simulink model "PD_SMC"  (R2017b)
settings: Solver=FixedStepAuto  StartTime=0.0  StopTime=100  FixedStep=0.01  RelTol=1e-3
values from neighbouring files (symbols this model uses):
  g = 9.81    [matlab.mat]    (also in thongsohethong.m = 9.8)
  L = 0.3    [thongsohethong.m]
  Mb = 7    [thongsohethong.m]
  Mw = 0.03    [matlab.mat]    (also in thongsohethong.m = 0.5)
  R = 1    [matlab.mat]    (also in thongsohethong.m = 0.07)
settings Model: Creator=DELL  LastModifiedBy=DELL

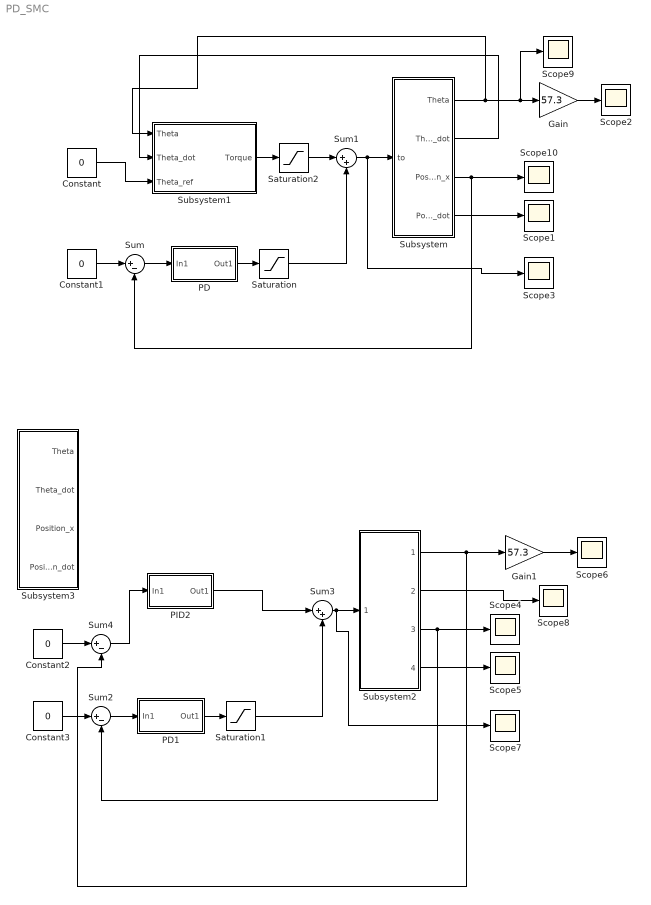
== system PD_SMC ==
  Constant{,1..3} (4 alike) : Constant  Value=0
  Gain : Gain  Gain=57.3
  Gain1 : Gain  Gain=57.3
  PD : Subsystem
  PD1 : Subsystem
  PID2 : Subsystem
  Saturation : Saturate  UpperLimit=0.25  LowerLimit=-0.25
  Saturation1 : Saturate
  Saturation2 : Saturate  UpperLimit=0.75  LowerLimit=-0.75
  Scope{1..10} (10 alike) : Scope
  Subsystem : Subsystem
  Subsystem1 : Subsystem
  Subsystem2 : Subsystem
  Subsystem3 : Subsystem
  Sum : Sum  Inputs=|+-
  Sum1 : Sum  Inputs=|++
  Sum2 : Sum  Inputs=|+-
  Sum3 : Sum  Inputs=|++
  Sum4 : Sum  Inputs=|+-
  wires:
  Subsystem/1(Theta) -> Subsystem1/1(Theta), Scope9/1, Gain/1
  Subsystem/2(Theta_dot) -> Subsystem1/2(Theta_dot)
  Subsystem/3(Position_x) -> Scope10/1, Sum/2
  Subsystem/4(Position_dot) -> Scope1/1
  Constant/1 -> Subsystem1/3(Theta_ref)
  Constant1/1 -> Sum/1
  Sum/1 -> PD/1(In1)
  PD/1(Out1) -> Saturation/1
  Saturation/1 -> Sum1/2
  Gain/1 -> Scope2/1
  Subsystem1/1(Torque) -> Saturation2/1
  PID2/1(Out1) -> Sum3/1
  PD1/1(Out1) -> Saturation1/1
  Sum2/1 -> PD1/1(In1)
  Sum3/1 -> Scope7/1, Subsystem2/1(Moment_motor)
  Constant3/1 -> Sum2/1
  Subsystem2/4(Position_dot) -> Scope5/1
  Subsystem2/1(Theta) -> Sum4/2, Gain1/1
  Saturation1/1 -> Sum3/2
  Subsystem2/3(Position_x) -> Sum2/2, Scope4/1
  Gain1/1 -> Scope6/1
  Constant2/1 -> Sum4/1
  Sum4/1 -> PID2/1(In1)
  Subsystem2/2(Theta_dot) -> Scope8/1
  Sum1/1 -> Scope3/1, Subsystem/1(to)
  Saturation2/1 -> Sum1/1

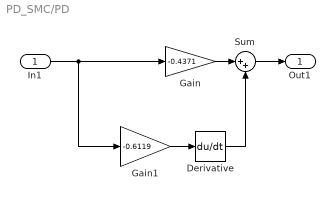
== system PD_SMC/PD ==
  In1 : Inport
  Derivative : Derivative
  Gain : Gain  Gain=-0.4371
  Gain1 : Gain  Gain=-0.6119
  Sum : Sum  Inputs=|++
  Out1 : Outport
  wires:
  In1/1 -> Gain1/1, Gain/1
  Gain1/1 -> Derivative/1
  Gain/1 -> Sum/1
  Sum/1 -> Out1/1
  Derivative/1 -> Sum/2

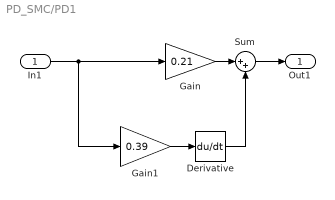
== system PD_SMC/PD1 ==
  In1 : Inport
  Derivative : Derivative
  Gain : Gain  Gain=0.21
  Gain1 : Gain  Gain=0.39
  Sum : Sum  Inputs=|++
  Out1 : Outport
  wires:
  In1/1 -> Gain1/1, Gain/1
  Gain1/1 -> Derivative/1
  Gain/1 -> Sum/1
  Sum/1 -> Out1/1
  Derivative/1 -> Sum/2

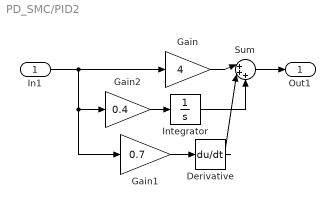
== system PD_SMC/PID2 ==
  In1 : Inport
  Derivative : Derivative
  Gain : Gain  Gain=4
  Gain1 : Gain  Gain=0.7
  Gain2 : Gain  Gain=0.4
  Integrator : Integrator
  Sum : Sum  Inputs=|+++
  Out1 : Outport
  wires:
  Derivative/1 -> Sum/2
  Sum/1 -> Out1/1
  Gain/1 -> Sum/1
  Gain1/1 -> Derivative/1
  In1/1 -> Gain/1, Gain2/1, Gain1/1
  Gain2/1 -> Integrator/1
  Integrator/1 -> Sum/3

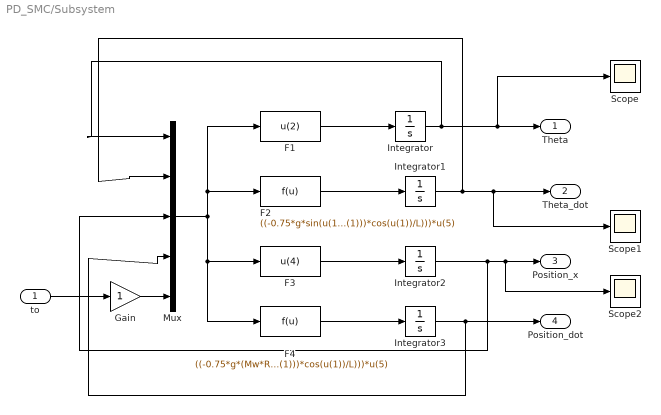
== system PD_SMC/Subsystem ==
  to : Inport
  F1 : Fcn  Expr=u(2)
  F2 : Fcn  Expr=((-0.75*g*sin(u(1))/L)/((0.75*((Mw*R+Mb*L*cos(u(1)))*cos(u(1)))/(2*Mw+Mb)*L)-1))+((0.75*Mb*L*sin(u(1))*cos(u(1))*(u(2)^2)/(2*Mw+Mb)*L)/((0.75*(Mw*R+Mb*L*cos(u(1)))*cos(u(1))/(2*Mw+Mb)*L)-1))+(((0.75*(Mw*R+Mb*L*cos(u(1)))*(1+(sin(u(1))^2)))+1/R)/(2*Mw+Mb-(0.75*(Mw*R+Mb*L*cos(u(1)))*cos(u(1))/L)))*u(5)
  F3 : Fcn  Expr=u(4)
  F4 : Fcn  Expr=((-0.75*g*(Mw*R+Mb*L*cos(u(1)))*sin(u(1)))/(2*Mw+Mb-(0.75*(Mw*R+Mb*L*cos(u(1)))*cos(u(1))/L)))+((Mb*L*sin(u(1))*(u(2)^2))/(2*Mw+Mb-(0.75*(Mw*R+Mb*L*cos(u(1)))*cos(u(1))/L)))+((0.75*(Mw*R+Mb*L*cos(u(1)))*(1+(sin(u(1))^2))+1/R)/(Mb*L^2)+(1/R)/(2*Mw+Mb-(0.75*(Mw*R+Mb*L*cos(u(1)))*cos(u(1))/L)))*u(5)
  Gain : Gain
  Integrator : Integrator  InitialCondition=0.3
  Integrator1 : Integrator
  Integrator2 : Integrator
  Integrator3 : Integrator
  Mux : Mux  Inputs=5
  Scope : Scope
  Scope1 : Scope
  Scope2 : Scope
  Theta : Outport
  Theta_dot : Outport  Port=2
  Position_x : Outport  Port=3
  Position_dot : Outport  Port=4
  wires:
  Gain/1 -> Mux/5
  F4/1 -> Integrator3/1
  Integrator3/1 -> Position_dot/1, Mux/4
  Integrator2/1 -> Mux/3, Position_x/1, Scope2/1
  Integrator/1 -> Theta/1, Scope/1, Mux/1
  F3/1 -> Integrator2/1
  F1/1 -> Integrator/1
  F2/1 -> Integrator1/1
  Integrator1/1 -> Theta_dot/1, Scope1/1, Mux/2
  Mux/1 -> F4/1, F3/1, F2/1, F1/1
  to/1 -> Gain/1

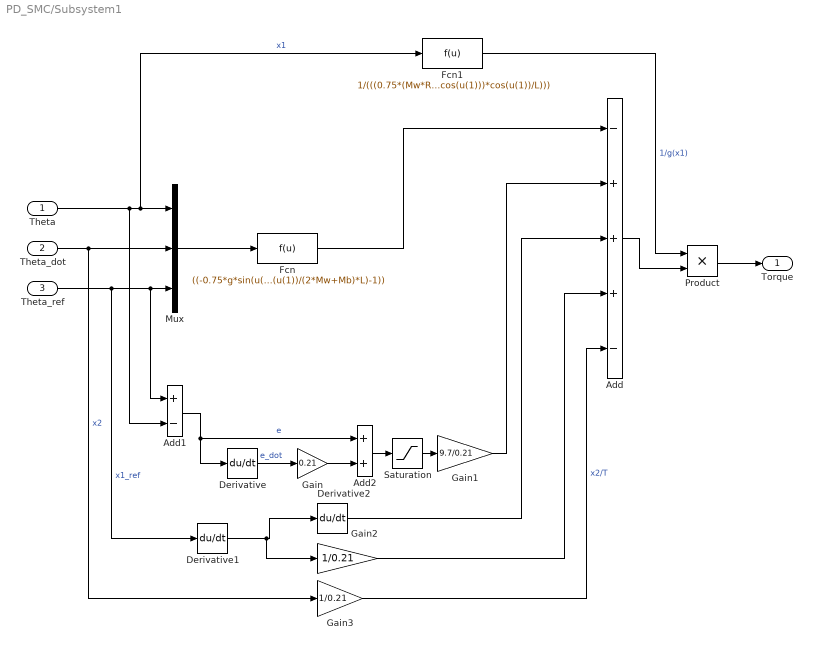
== system PD_SMC/Subsystem1 ==
  Theta : Inport
  Theta_dot : Inport  Port=2
  Theta_ref : Inport  Port=3
  Add : Sum  Inputs=-+++-
  Add1 : Sum  Inputs=+-
  Add2 : Sum
  Derivative : Derivative
  Derivative1 : Derivative
  Derivative2 : Derivative
  Fcn : Fcn  Expr=((-0.75*g*sin(u(1))/L)/((0.75*((Mw*R+Mb*L*cos(u(1)))*cos(u(1)))/(2*Mw+Mb)*L)-1))+((0.75*Mb*L*sin(u(1))*cos(u(1))*(u(2)^2)/(2*Mw+Mb)*L)/((0.75*(Mw*R+Mb*L*cos(u(1)))*cos(u(1))/(2*Mw+Mb)*L)-1))
  Fcn1 : Fcn  Expr=1/(((0.75*(Mw*R+Mb*L*cos(u(1)))*(1+(sin(u(1))^2)))+1/R)/(2*Mw+Mb-(0.75*(Mw*R+Mb*L*cos(u(1)))*cos(u(1))/L)))
  Gain : Gain  Gain=0.21
  Gain1 : Gain  Gain=9.7/0.21
  Gain2 : Gain  Gain=1/0.21
  Gain3 : Gain  Gain=1/0.21
  Mux : Mux  Inputs=3
  Product : Product
  Saturation : Saturate  UpperLimit=0.4  LowerLimit=-0.4
  Torque : Outport
  wires:
  Theta_dot/1 -> Gain3/1, Mux/2  "x2"
  Theta/1 -> Fcn1/1, Mux/1, Add1/2  "x1"
  Theta_ref/1 -> Derivative1/1, Add1/1, Mux/3  "x1_ref"
  Add1/1 -> Derivative/1, Add2/1  "e"
  Derivative/1 -> Gain/1  "e_dot"
  Gain/1 -> Add2/2
  Add2/1 -> Saturation/1
  Saturation/1 -> Gain1/1
  Gain1/1 -> Add/2
  Derivative1/1 -> Gain2/1, Derivative2/1
  Derivative2/1 -> Add/3
  Gain2/1 -> Add/4
  Gain3/1 -> Add/5  "x2/T"
  Mux/1 -> Fcn/1
  Fcn/1 -> Add/1
  Fcn1/1 -> Product/1  "1/g(x1)"
  Add/1 -> Product/2
  Product/1 -> Torque/1

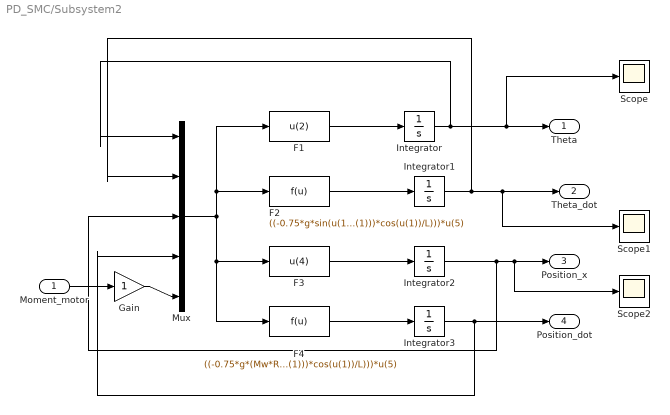
== system PD_SMC/Subsystem2 ==
  Moment_motor : Inport
  F1 : Fcn  Expr=u(2)
  F2 : Fcn  Expr=((-0.75*g*sin(u(1))/L)/((0.75*((Mw*R+Mb*L*cos(u(1)))*cos(u(1)))/(2*Mw+Mb)*L)-1))+((0.75*Mb*L*sin(u(1))*cos(u(1))*(u(2)^2)/(2*Mw+Mb)*L)/((0.75*(Mw*R+Mb*L*cos(u(1)))*cos(u(1))/(2*Mw+Mb)*L)-1))+(((0.75*(Mw*R+Mb*L*cos(u(1)))*(1+(sin(u(1))^2)))+1/R)/(2*Mw+Mb-(0.75*(Mw*R+Mb*L*cos(u(1)))*cos(u(1))/L)))*u(5)
  F3 : Fcn  Expr=u(4)
  F4 : Fcn  Expr=((-0.75*g*(Mw*R+Mb*L*cos(u(1)))*sin(u(1)))/(2*Mw+Mb-(0.75*(Mw*R+Mb*L*cos(u(1)))*cos(u(1))/L)))+((Mb*L*sin(u(1))*(u(2)^2))/(2*Mw+Mb-(0.75*(Mw*R+Mb*L*cos(u(1)))*cos(u(1))/L)))+((0.75*(Mw*R+Mb*L*cos(u(1)))*(1+(sin(u(1))^2))+1/R)/(Mb*L^2)+(1/R)/(2*Mw+Mb-(0.75*(Mw*R+Mb*L*cos(u(1)))*cos(u(1))/L)))*u(5)
  Gain : Gain
  Integrator : Integrator  InitialCondition=0.01
  Integrator1 : Integrator
  Integrator2 : Integrator
  Integrator3 : Integrator
  Mux : Mux  Inputs=5
  Scope : Scope
  Scope1 : Scope
  Scope2 : Scope
  Theta : Outport
  Theta_dot : Outport  Port=2
  Position_x : Outport  Port=3
  Position_dot : Outport  Port=4
  wires:
  Gain/1 -> Mux/5
  F4/1 -> Integrator3/1
  Moment_motor/1 -> Gain/1
  Integrator3/1 -> Position_dot/1, Mux/4
  Integrator2/1 -> Mux/3, Position_x/1, Scope2/1
  Integrator/1 -> Theta/1, Scope/1, Mux/1
  F3/1 -> Integrator2/1
  F1/1 -> Integrator/1
  F2/1 -> Integrator1/1
  Integrator1/1 -> Theta_dot/1, Scope1/1, Mux/2
  Mux/1 -> F4/1, F3/1, F2/1, F1/1

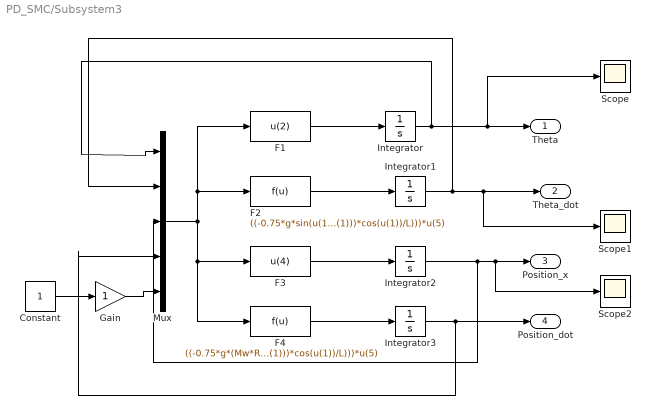
== system PD_SMC/Subsystem3 ==
  Constant : Constant
  F1 : Fcn  Expr=u(2)
  F2 : Fcn  Expr=((-0.75*g*sin(u(1))/L)/((0.75*((Mw*R+Mb*L*cos(u(1)))*cos(u(1)))/(2*Mw+Mb)*L)-1))+((0.75*Mb*L*sin(u(1))*cos(u(1))*(u(2)^2)/(2*Mw+Mb)*L)/((0.75*(Mw*R+Mb*L*cos(u(1)))*cos(u(1))/(2*Mw+Mb)*L)-1))+(((0.75*(Mw*R+Mb*L*cos(u(1)))*(1+(sin(u(1))^2)))+1/R)/(2*Mw+Mb-(0.75*(Mw*R+Mb*L*cos(u(1)))*cos(u(1))/L)))*u(5)
  F3 : Fcn  Expr=u(4)
  F4 : Fcn  Expr=((-0.75*g*(Mw*R+Mb*L*cos(u(1)))*sin(u(1)))/(2*Mw+Mb-(0.75*(Mw*R+Mb*L*cos(u(1)))*cos(u(1))/L)))+((Mb*L*sin(u(1))*(u(2)^2))/(2*Mw+Mb-(0.75*(Mw*R+Mb*L*cos(u(1)))*cos(u(1))/L)))+((0.75*(Mw*R+Mb*L*cos(u(1)))*(1+(sin(u(1))^2))+1/R)/(Mb*L^2)+(1/R)/(2*Mw+Mb-(0.75*(Mw*R+Mb*L*cos(u(1)))*cos(u(1))/L)))*u(5)
  Gain : Gain
  Integrator{,1..3} (4 alike) : Integrator
  Mux : Mux  Inputs=5
  Scope : Scope
  Scope1 : Scope
  Scope2 : Scope
  Theta : Outport
  Theta_dot : Outport  Port=2
  Position_x : Outport  Port=3
  Position_dot : Outport  Port=4
  wires:
  Gain/1 -> Mux/5
  F4/1 -> Integrator3/1
  Integrator3/1 -> Position_dot/1, Mux/4
  Integrator2/1 -> Mux/3, Position_x/1, Scope2/1
  Integrator/1 -> Theta/1, Scope/1, Mux/1
  F3/1 -> Integrator2/1
  F1/1 -> Integrator/1
  F2/1 -> Integrator1/1
  Integrator1/1 -> Theta_dot/1, Scope1/1, Mux/2
  Mux/1 -> F2/1, F1/1, F4/1, F3/1
  Constant/1 -> Gain/1
